simulink model "lab2_spectrometer_simulink_CRD"  (R2025b)
settings: Solver=FixedStepDiscrete  StartTime=0.0  StopTime=0.000001  RelTol=1e-3
undefined symbols (not defined in the file): Add, Fs, N, Shift, Ts
libraries: dsphdlsigops2 x2, dsphdlmathfun2 x1, dsphdlxfrm2 x1
settings Model: Creator=caleb  LastModifiedBy=caleb

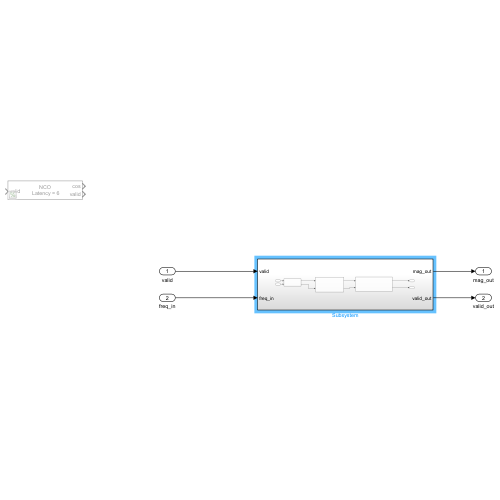
[thumbnail: Simulink's stored preview of the top-level diagram]
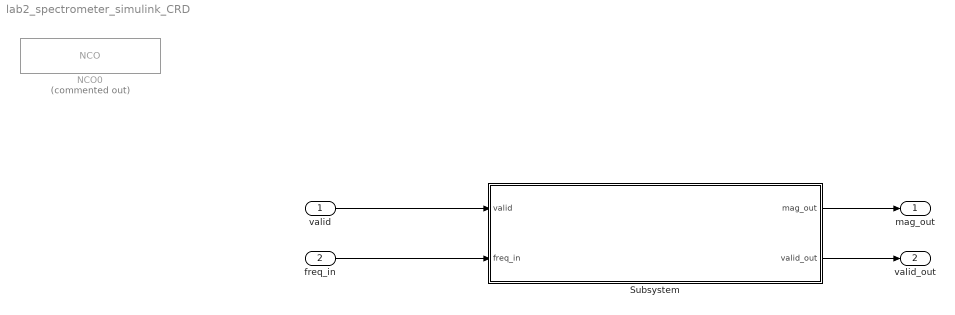
== system lab2_spectrometer_simulink_CRD ==
  valid : Inport  OutDataTypeStr=boolean
  freq_in : Inport  Port=2
  NCO0 : dsphdlsigops2/NCO  Commented=on  PhaseIncrementSource=Property  PhaseIncrement=phIncr4  PhaseOffsetSource=Property  PhaseOffset=phOff  DitherSource=Property  NumDitherBits=ditherBits  SamplesPerFrame=1  LUTCompress=off  ResetAction=off  Waveform=Cosine  PhasePort=off  SimulateUsing=Code generation  AccumulatorWL=N  PhaseQuantization=on  NumQuantizerAccumulatorBits=Q  OutputDataType=Binary point scaling  OutputWL=16  OutputFL=14
  Subsystem : Subsystem
  mag_out : Outport  VectorParamsAs1DForOutWhenUnconnected=off
  valid_out : Outport  Port=2  VectorParamsAs1DForOutWhenUnconnected=off
  wires:
  valid/1 -> Subsystem/1(valid)
  freq_in/1 -> Subsystem/2(freq_in)
  Subsystem/1(mag_out) -> mag_out/1
  Subsystem/2(valid_out) -> valid_out/1

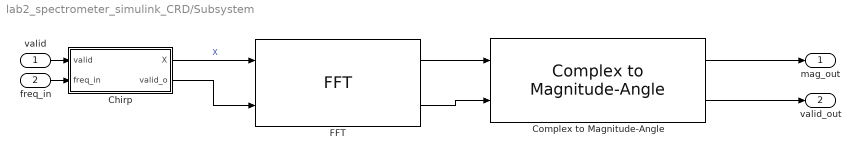
== system lab2_spectrometer_simulink_CRD/Subsystem ==
  valid : Inport
  freq_in : Inport  Port=2
  Chirp : Subsystem
  Complex to Magnitude-Angle : dsphdlmathfun2/Complex to Magnitude-Angle  NumIterationsSource=Auto  NumIterations=10  OutputFormat=Magnitude  AngleFormat=Normalized  ScaleOutput=on  ScalingMethod=Shift-Add  SimulateUsing=Code generation
  FFT : dsphdlxfrm2/FFT  Architecture=Streaming Radix 2^2  FFTLengthSource=Property  FFTLength=FFT_SIZE  FFTLengthMax=1024  ComplexMultiplication=Use 4 multipliers and 2 adders  BitReversedOutput=on  BitReversedInput=off  Normalize=off  SimulateUsing=Code generation  RoundingMethod=Floor  ResetInputPort=off  StartOutputPort=off  EndOutputPort=off
  mag_out : Outport
  valid_out : Outport  Port=2
  wires:
  FFT/1 -> Complex to Magnitude-Angle/1
  Complex to Magnitude-Angle/2 -> valid_out/1
  Chirp/2(valid_o) -> FFT/2
  valid/1 -> Chirp/1(valid)
  FFT/2 -> Complex to Magnitude-Angle/2
  Complex to Magnitude-Angle/1 -> mag_out/1
  Chirp/1(X) -> FFT/1  "X"
  freq_in/1 -> Chirp/2(freq_in)

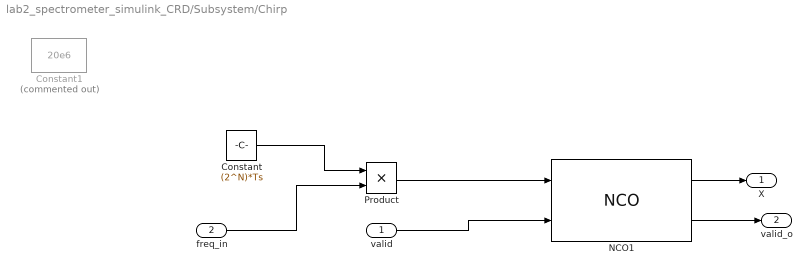
== system lab2_spectrometer_simulink_CRD/Subsystem/Chirp ==
  valid : Inport
  freq_in : Inport  Port=2
  Constant : Constant  Value=(2^N)*Ts  OutDataTypeStr=fixdt(0,16,10)  SampleTime=1/Fs
  Constant1 : Constant  Commented=on  Value=20e6
  NCO1 : dsphdlsigops2/NCO  PhaseIncrementSource=Input port  PhaseIncrement=phIncr  PhaseOffsetSource=Property  PhaseOffset=phOff  DitherSource=Property  NumDitherBits=ditherBits  SamplesPerFrame=1  LUTCompress=off  ResetAction=off  Waveform=Cosine  PhasePort=off  SimulateUsing=Code generation  AccumulatorWL=N  PhaseQuantization=on  NumQuantizerAccumulatorBits=Q  OutputDataType=Binary point scaling  OutputWL=16  OutputFL=14
  Product : Product  OutDataTypeStr=uint32  LockScale=on
  X : Outport
  valid_o : Outport  Port=2
  wires:
  Constant/1 -> Product/1
  valid/1 -> NCO1/2
  NCO1/2 -> valid_o/1
  NCO1/1 -> X/1
  Product/1 -> NCO1/1
  freq_in/1 -> Product/2
